simulink subsystem "Dead_Reckoning_3DoF"  (R2024b)
settings: Solver=VariableStepAuto  StartTime=0.0  StopTime=10.0  RelTol=1e-3
undefined symbols (not defined in the file or in its folder): filter_update_time, fractalcoef, lla_ref, x0
libraries: sensorgpslib x1, mspsensorlib x1
settings Model: Creator=thatf  LastModifiedBy=thatf

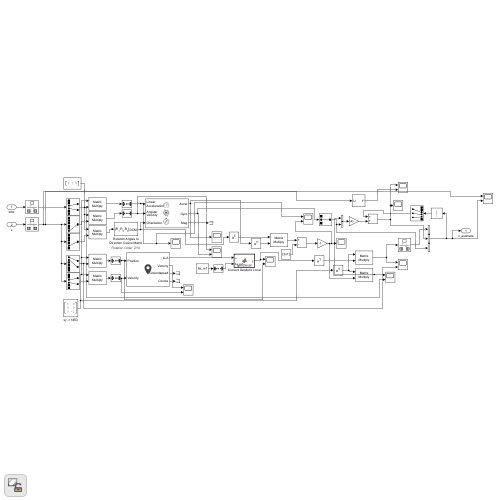
[thumbnail: Simulink's stored preview of the top-level diagram]
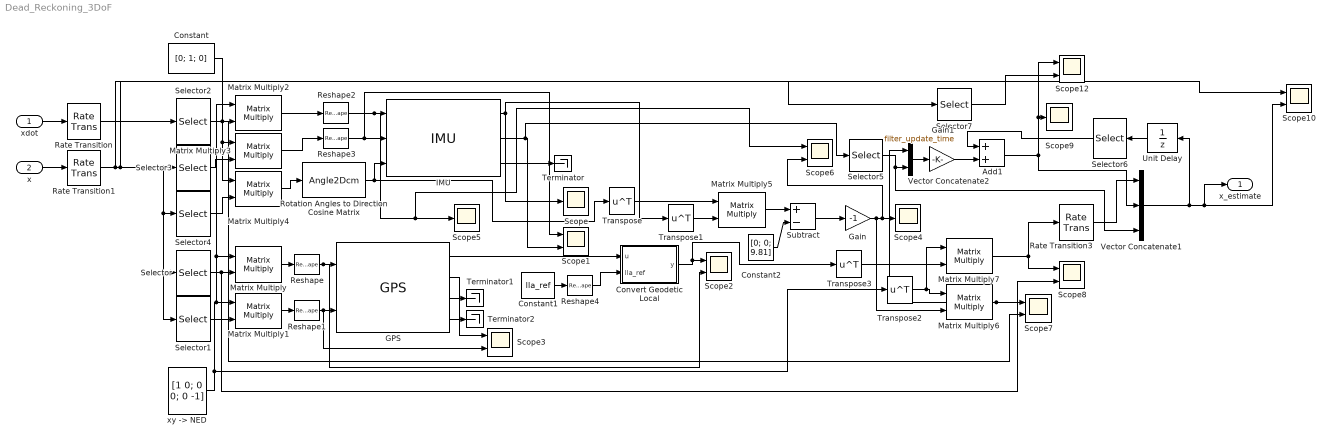
== system Dead_Reckoning_3DoF ==
  xdot : Inport
  x : Inport  Port=2
  Add1 : Sum
  Constant : Constant  Value=[0; 1; 0]
  Constant1 : Constant  Value=lla_ref
  Constant2 : Constant  Value=[0; 0; 9.81]
  Convert Geodetic Local : MATLAB Function  TreatAsAtomicUnit=on
  GPS : sensorgpslib/GPS  DispRefFrame=NED  PositionInputFormat=Local  ReferenceLocation=lla_ref  HorizontalPositionAccuracy=0.5  VerticalPositionAccuracy=1  VelocityAccuracy=0.1  DecayFactor=0.999  SeedDouble=67  SimulateUsing=Interpreted execution
  Gain : Gain  Gain=-1
  Gain1 : Gain  Gain=filter_update_time
  IMU : mspsensorlib/IMU  DispRefFrame=NED  TemperaturePort=off  Temperature=25  MagneticFieldPort=off  MagneticFieldNED=[ 27.5550, -2.4169, -16.0849 ]  MagneticFieldENU=[ -2.4169, 27.5550, 16.0849 ]  SeedDouble=67  SimulateUsing=Interpreted execution  AccelParamsMeasurementRange=Inf  AccelParamsResolution=0  AccelParamsConstantBias=[ 0, 0, 0 ]  AccelParamsAxesMisalignment=[ 100, 0, 0; 0, 100, 0; 0, 0, 100 ]  AccelParamsNoiseDensity=[ 0.1, 0.1, 0.1 ]  AccelParamsBiasInstability=[ 0, 0, 0 ]  AccelParamsBiasInstabilityNumerator=fractalcoef().Numerator  AccelParamsBiasInstabilityDenominator=fractalcoef().Denominator  AccelParamsRandomWalk=[ 0.1, 0.1, 0.1 ]  AccelParamsNoiseType=double-sided  AccelParamsTemperatureBias=[ 0, 0, 0 ]  AccelParamsTemperatureScaleFactor=[ 0, 0, 0 ]  GyroParamsMeasurementRange=Inf  GyroParamsResolution=0  GyroParamsConstantBias=[ 0, 0, 0 ]  GyroParamsAxesMisalignment=[ 100, 0, 0; 0, 100, 0; 0, 0, 100 ]  GyroParamsAccelerationBias=[ 0, 0, 0 ]  GyroParamsNoiseDensity=[ 0.0002, 0.0002, 0.0002 ]  GyroParamsBiasInstability=[ 0, 0, 0 ]  GyroParamsBiasInstabilityNumerator=fractalcoef().Numerator  GyroParamsBiasInstabilityDenominator=fractalcoef().Denominator  GyroParamsRandomWalk=[ 0.0002, 0.0002, 0.0002 ]  GyroParamsNoiseType=double-sided  GyroParamsTemperatureBias=[ 0, 0, 0 ]  GyroParamsTemperatureScaleFactor=[ 0, 0, 0 ]  MagParamsMeasurementRange=Inf  MagParamsResolution=0  MagParamsConstantBias=[ 0, 0, 0 ]  MagParamsAxesMisalignment=[ 100, 0, 0; 0, 100, 0; 0, 0, 100 ]  MagParamsNoiseDensity=[ 0, 0, 0 ]  MagParamsBiasInstability=[ 0, 0, 0 ]  MagParamsBiasInstabilityNumerator=fractalcoef().Numerator  MagParamsBiasInstabilityDenominator=fractalcoef().Denominator  MagParamsRandomWalk=[ 0, 0, 0 ]  MagParamsNoiseType=double-sided  MagParamsTemperatureBias=[ 0, 0, 0 ]  MagParamsTemperatureScaleFactor=[ 0, 0, 0 ]
  Matrix Multiply{,1..7} (8 alike) : Product  Multiplication=Matrix(*)
  Rate Transition : RateTransition  OutPortSampleTime=filter_update_time
  Rate Transition1 : RateTransition  InitialCondition=x0  OutPortSampleTime=filter_update_time
  Rate Transition3 : RateTransition  InitialCondition=[x0(1), x0(2)]  OutPortSampleTime=0.05
  Reshape{,1..4} (5 alike) : Reshape  OutputDimensionality=Row vector (2-D)
  Rotation Angles to Direction Cosine Matrix : Angle2Dcm
      settings: AttributesFormatString=Rotation Order: %<rotationOrder>
  Scope{,4..5,9} (4 alike) : Scope
  Scope{1..3,6..8,10,12} (8 alike) : Scope  NumInputPorts=2
  Selector : Selector  InputPortWidth=6  IndexOptions=Index vector (dialog)  Indices=[1 2]  OutputSizes=1
  Selector1 : Selector  InputPortWidth=6  IndexOptions=Index vector (dialog)  Indices=[3 4]  OutputSizes=1
  Selector2 : Selector  InputPortWidth=6  IndexOptions=Index vector (dialog)  Indices=[3 4]  OutputSizes=1
  Selector3 : Selector  InputPortWidth=6  IndexOptions=Index vector (dialog)  Indices=[6]  OutputSizes=1
  Selector4 : Selector  InputPortWidth=6  IndexOptions=Index vector (dialog)  Indices=[5]  OutputSizes=1
  Selector5 : Selector  InputPortWidth=3  IndexOptions=Index vector (dialog)  Indices=[2]  OutputSizes=1
  Selector6 : Selector  InputPortWidth=6  IndexOptions=Index vector (dialog)  Indices=[3 4 5]  OutputSizes=1
  Selector7 : Selector  InputPortWidth=6  IndexOptions=Index vector (dialog)  Indices=[3 4 6]  OutputSizes=1
  Subtract : Sum  Inputs=+-
  Terminator : Terminator
  Terminator1 : Terminator
  Terminator2 : Terminator
  Transpose{,1..3} (4 alike) : Math  Operator=transpose
  Unit Delay : UnitDelay  InitialCondition=x0'  SampleTime=-1  HasFrameUpgradeWarning=on
  Vector Concatenate1 : Concatenate  NumInputs=3
  Vector Concatenate2 : Concatenate
  "xy -> NED" : Constant  Value=[1 0; 0 0; 0 -1]
  x_estimate : Outport
  wires:
  Convert Geodetic Local/1(y) -> Scope2/1, Transpose3/1
  Reshape1/1 -> GPS/2, Scope3/2
  GPS/3 -> Terminator1/1
  Matrix Multiply/1 -> Reshape/1
  Rotation Angles to Direction Cosine Matrix/1 -> IMU/3, Transpose/1
  Reshape/1 -> GPS/1, Scope2/2
  IMU/2 -> Scope1/2, Selector5/1
  Selector/1 -> Matrix Multiply/2, Scope8/2
  Matrix Multiply1/1 -> Reshape1/1
  Selector3/1 -> Matrix Multiply3/2
  Transpose3/1 -> Matrix Multiply7/2
  Matrix Multiply6/1 -> Scope7/1, Vector Concatenate2/1
  Gain/1 -> Scope4/1, Scope6/2, Matrix Multiply6/2
  Matrix Multiply2/1 -> Reshape2/1
  Constant1/1 -> Reshape4/1
  Reshape3/1 -> IMU/2, Scope1/1
  Transpose2/1 -> Matrix Multiply6/1, Matrix Multiply7/1
  Vector Concatenate1/1 -> Scope10/2, x_estimate/1, Unit Delay/1
  Rate Transition/1 -> Selector2/1
  GPS/1 -> Convert Geodetic Local/1(u)
  IMU/1 -> Transpose1/1, Scope/1
  GPS/4 -> Terminator2/1
  Reshape4/1 -> Convert Geodetic Local/2(lla_ref)
  xdot/1 -> Rate Transition/1
  Selector5/1 -> Vector Concatenate2/2, Vector Concatenate1/3
  Reshape2/1 -> IMU/1, Scope5/1, Scope6/1
  x/1 -> Rate Transition1/1
  Add1/1 -> Scope9/1, Scope12/1, Vector Concatenate1/2
  Selector4/1 -> Matrix Multiply4/2
  Matrix Multiply7/1 -> Rate Transition3/1, Scope8/1
  Unit Delay/1 -> Selector6/1
  Constant/1 -> Matrix Multiply3/1, Matrix Multiply4/1
  Transpose/1 -> Matrix Multiply5/1
  Selector1/1 -> Matrix Multiply1/2
  Gain1/1 -> Add1/2
  Matrix Multiply4/1 -> Rotation Angles to Direction Cosine Matrix/1
  "xy -> NED"/1 -> Matrix Multiply1/1, Matrix Multiply2/1, Matrix Multiply/1, Transpose2/1
  Subtract/1 -> Gain/1
  IMU/3 -> Terminator/1
  Selector6/1 -> Add1/1
  Rate Transition3/1 -> Vector Concatenate1/1
  Matrix Multiply3/1 -> Reshape3/1
  Transpose1/1 -> Matrix Multiply5/2
  Constant2/1 -> Subtract/2
  Selector2/1 -> Matrix Multiply2/2, Scope7/2
  Selector7/1 -> Scope12/2
  GPS/2 -> Scope3/1
  Matrix Multiply5/1 -> Subtract/1
  Vector Concatenate2/1 -> Gain1/1
  Rate Transition1/1 -> Selector3/1, Selector4/1, Selector/1, Selector1/1, Scope10/1, Selector7/1

== matlab function Dead_Reckoning_3DoF/Convert Geodetic Local ==
  data: u input; y output; lla_ref input
function y = geo2local(u, lla_ref)

y = lla2ned(u,lla_ref,"ellipsoid");

end
